simulink model "simulink_multiple_step_ODE_PID"  (R2023a)
settings: Solver=ode45  StartTime=0.0  StopTime=15000  RelTol=1e-3
libraries: slpidlib x1
settings Model: Creator=USER  LastModifiedBy=USER

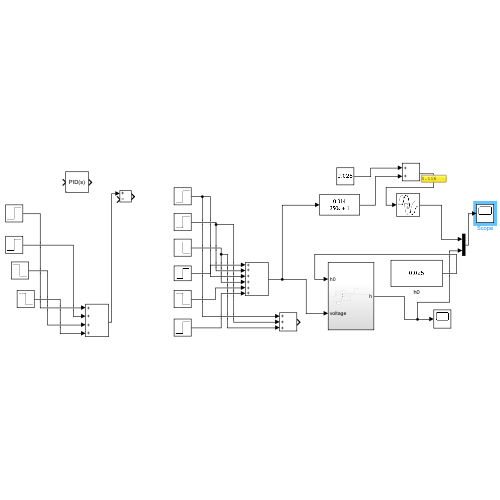
[thumbnail: Simulink's stored preview of the top-level diagram]
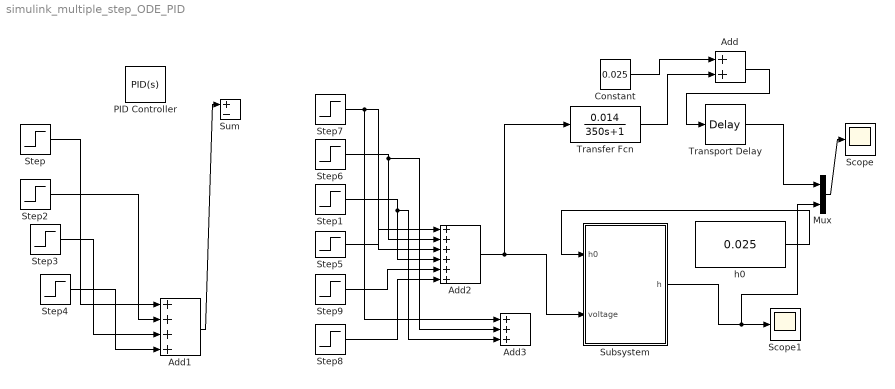
== system simulink_multiple_step_ODE_PID ==
  Add : Sum
  Add1 : Sum  Inputs=++++
  Add2 : Sum  Inputs=++++++
  Add3 : Sum  Inputs=+++
  Constant : Constant  Value=0.025
  Mux : Mux  Inputs=2
  PID Controller : slpidlib/PID Controller  Controller=PID  Form=Parallel  TimeDomain=Continuous-time  UseExternalTs=off  SampleTime=-1  IntegratorMethod=Forward Euler  FilterMethod=Forward Euler  ControllerParametersSource=internal  P=1  I=10  UseKiTs=off  D=0  N=100  UseFilter=on  TunerSelectOption=Transfer Function Based (PID Tuner App)  InitialConditionSource=internal  InitialConditionForIntegrator=0  InitialConditionForFilter=0  DifferentiatorICPrevScaledInput=0  ExternalReset=none  TrackingMode=off  Kt=1  LimitOutput=off  SatLimitsSource=internal  UpperSaturationLimit=inf  LowerSaturationLimit=-inf  LinearizeAsGain=on  AntiWindupMode=none  Kb=1  LimitIntegrator=off  UpperIntegratorSaturationLimit=inf  LowerIntegratorSaturationLimit=-inf  POutMin=[]  POutMax=[]  IOutMin=[]  IOutMax=[]  DOutMin=[]  DOutMax=[]  NOutMin=[]  NOutMax=[]  SumOutMin=[]  SumOutMax=[]  SaturationOutMin=[]  SaturationOutMax=[]  PParamMin=[]  PParamMax=[]  IParamMin=[]  IParamMax=[]  DParamMin=[]  DParamMax=[]  NParamMin=[]  NParamMax=[]  KbParamMin=[]  KbParamMax=[]  KtParamMin=[]  KtParamMax=[]  KbOutMin=[]  KbOutMax=[]  KtOutMin=[]  KtOutMax=[]  IntegratorOutMin=[]  IntegratorOutMax=[]  FilterOutMin=[]  FilterOutMax=[]  SumI1OutMin=[]  SumI1OutMax=[]  SumI2OutMin=[]  SumI2OutMax=[]  SumI3OutMin=[]  SumI3OutMax=[]  SumI4OutMin=[]  SumI4OutMax=[]  SumDOutMin=[]  SumDOutMax=[]  DifferentiatorOutMin=[]  DifferentiatorOutMax=[]  FilterDiffOutCoefMin=[]  FilterDiffOutCoefMax=[]  ReciprocalOutMin=[]  ReciprocalOutMax=[]  SumDenOutMin=[]  SumDenOutMax=[]  SumNumOutMin=[]  SumNumOutMax=[]  DivideOutMin=[]  DivideOutMax=[]  UdiffTsProdOutMin=[]  UdiffTsProdOutMax=[]  NTsProdOutMin=[]  NTsProdOutMax=[]  UintegralTsProdOutMin=[]  UintegralTsProdOutMax=[]  UngainTsProdOutMin=[]  UngainTsProdOutMax=[]  ClampingZeroOutDataTypeStr=Inherit: Inherit via back propagation  ClampingZeroOutMin=[]  ClampingZeroOutMax=[]  FilterDenConstantOutDataTypeStr=Inherit: Inherit via back propagation  FilterDenConstantOutMin=[]  FilterDenConstantOutMax=[]  PCopyOutDataTypeStr=Inherit: Inherit via back propagation  PCopyOutMin=[]  PCopyOutMax=[]  NCopyOutDataTypeStr=Inherit: Inherit via back propagation  NCopyOutMin=[]  NCopyOutMax=[]  IntegratorContinuousStateAttributes=''  IntegratorStateMustResolveToSignalObject=off  IntegratorRTWStateStorageClass=Auto  FilterContinuousStateAttributes=''  FilterStateMustResolveToSignalObject=off  FilterRTWStateStorageClass=Auto  ParallelPVariant=InternalParameters  IdealPVariant=Disabled  IVariant=InternalParameters  DVariant=InternalParameters  IntegratorVariant=Continuous  SatVariant=Disabled  AWVariant=Passthrough  PCopyVariant=Disabled  TRVariant=Disabled  FdbkBlocksVariant=Forward  IdealPFdbkVariant=Disabled  SatFdbkVariant=Disabled  DerivativeFilterVariant=ContFilter  NVariant=InternalParameters  NCopyVariant=Disabled  FilterICVariant=InternalICsFilter  IntegratorICVariant=InternalICs  ExternalResetVariant=Disabled  TRSumVariant=Passthrough  SumFdbkVariant=Disabled  SumVariant=Sum_PID  TsampFilterVariant=InternalTs  TsampNgainVariant=Passthrough  TsampIntegralVariant=Disabled_SignalSpec  ExternalSaturationOutDataTypeStr=Inherit: Same as second input
  Scope : Scope
  Scope1 : Scope
  Step : Step  Time=100  Before=0.025  After=0.05  SampleTime=0.01
  Step1 : Step  Time=7000  After=-3  SampleTime=0.01
  Step2 : Step  Time=2500  After=0.05  SampleTime=0
  Step3 : Step  Time=5000  After=-0.02  SampleTime=0
  Step4 : Step  Time=7500  After=-0.03  SampleTime=0
  Step5 : Step  Time=8500  After=2  SampleTime=0.01
  Step6 : Step  Time=4000  After=2  SampleTime=0.01
  Step7 : Step  Time=0  After=5  SampleTime=0.01
  Step8 : Step  Time=12500  After=4  SampleTime=0.01
  Step9 : Step  Time=10000  After=-3.5  SampleTime=0.01
  Subsystem : Subsystem
  Sum : Sum  Inputs=+-
  Transfer Fcn : TransferFcn  Numerator=[0.014]  Denominator=[350 1]
  Transport Delay : TransportDelay  DelayTime=100  InitialOutput=0.025
  h0 : Constant  Value=0.025
  wires:
  Subsystem/1(h) -> Mux/2, Scope1/1
  Step/1 -> Add1/1
  Step2/1 -> Add1/2
  Step3/1 -> Add1/3
  Step4/1 -> Add1/4
  Add1/1 -> Sum/1
  h0/1 -> Subsystem/1(h0)
  Step1/1 -> Add3/3, Add2/4
  Step5/1 -> Add2/1
  Step9/1 -> Add2/5
  Step8/1 -> Add2/6
  Step7/1 -> Add3/1, Add2/3
  Step6/1 -> Add3/2, Add2/2
  Mux/1 -> Scope/1
  Constant/1 -> Add/1
  Transfer Fcn/1 -> Add/2
  Add/1 -> Transport Delay/1
  Transport Delay/1 -> Mux/1
  Add2/1 -> Transfer Fcn/1, Subsystem/2(voltage)

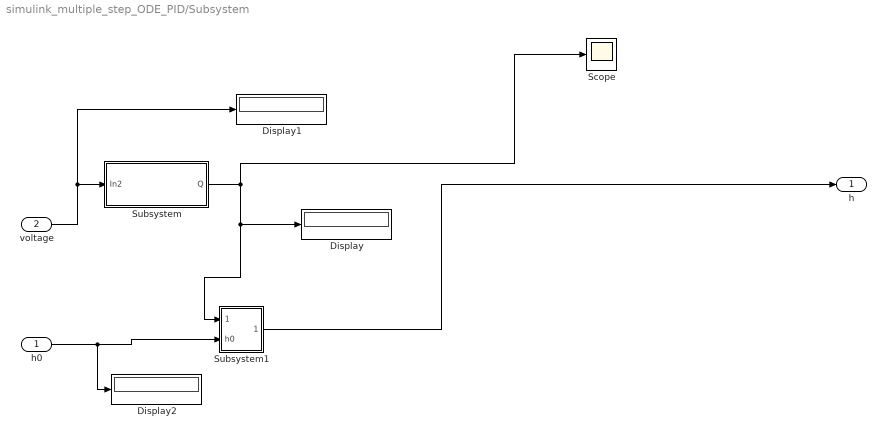
== system simulink_multiple_step_ODE_PID/Subsystem ==
  h0 : Inport
  voltage : Inport  Port=2
  Display : Display
  Display1 : Display
  Display2 : Display
  Scope : Scope
  Subsystem : Subsystem
  Subsystem1 : Subsystem
  h : Outport
  wires:
  Subsystem/1(Q) -> Subsystem1/1(In1), Display/1, Scope/1
  h0/1 -> Display2/1, Subsystem1/2(h0)
  Subsystem1/1(Out1) -> h/1
  voltage/1 -> Display1/1, Subsystem/1(In2)

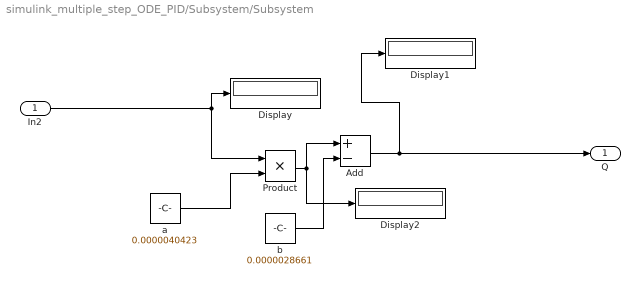
== system simulink_multiple_step_ODE_PID/Subsystem/Subsystem ==
  In2 : Inport
  Add : Sum  Inputs=+-
  Display : Display
  Display1 : Display
  Display2 : Display
  Product : Product
  a : Constant  Value=0.0000040423
  b : Constant  Value=0.0000028661
  Q : Outport
  wires:
  a/1 -> Product/2
  Product/1 -> Add/1, Display2/1
  b/1 -> Add/2
  Add/1 -> Display1/1, Q/1
  In2/1 -> Product/1, Display/1

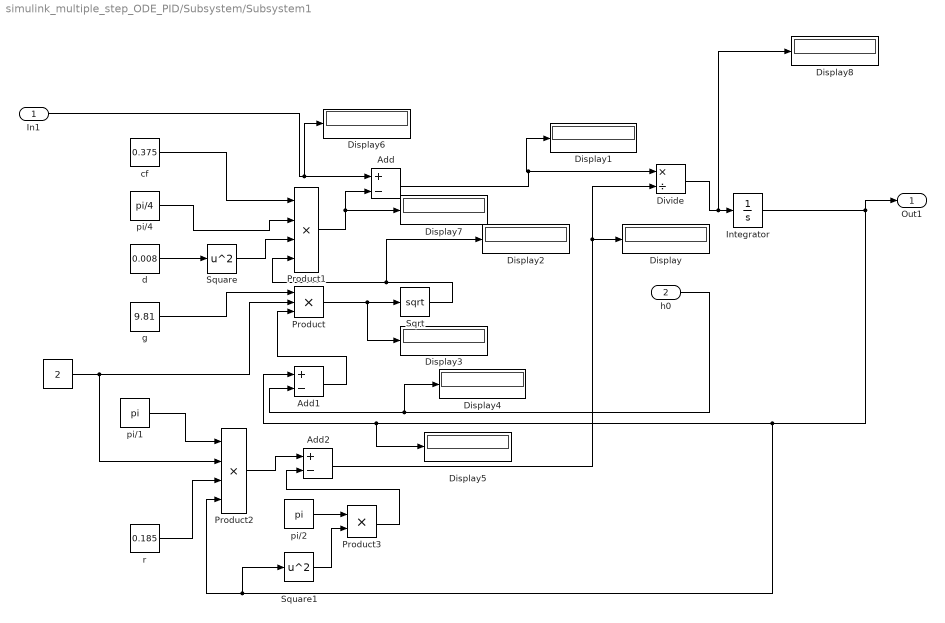
== system simulink_multiple_step_ODE_PID/Subsystem/Subsystem1 ==
  In1 : Inport
  h0 : Inport  Port=2
  " " : Constant  Value=2
  Add : Sum  Inputs=+-
  Add1 : Sum  Inputs=+-
  Add2 : Sum  Inputs=+-
  Display{,1..8} (9 alike) : Display
  Divide : Product  Inputs=*/
  Integrator : Integrator  InitialCondition=0.025
  Product : Product  Inputs=3
  Product1 : Product  Inputs=4
  Product2 : Product  Inputs=4
  Product3 : Product
  Sqrt : Sqrt
  Square : Math  Operator=square
  Square1 : Math  Operator=square
  cf : Constant  Value=0.375
  d : Constant  Value=0.008
  g : Constant  Value=9.81
  pi/1 : Constant  Value=pi
  pi/2 : Constant  Value=pi
  pi/4 : Constant  Value=pi/4
  r : Constant  Value=0.185
  Out1 : Outport
  wires:
  pi/1/1 -> Product2/1
  Add1/1 -> Product/3
  Product1/1 -> Display7/1, Add/2
  Divide/1 -> Display8/1, Integrator/1
  Product3/1 -> Add2/2
  " "/1 -> Product2/2, Product/2
  cf/1 -> Product1/1
  r/1 -> Product2/3
  Sqrt/1 -> Display2/1, Product1/4
  Square/1 -> Product1/3
  Product2/1 -> Add2/1
  pi/4/1 -> Product1/2
  h0/1 -> Display4/1, Add1/2
  g/1 -> Product/1
  d/1 -> Square/1
  Product/1 -> Display3/1, Sqrt/1
  Add/1 -> Divide/1, Display1/1
  Square1/1 -> Product3/2
  In1/1 -> Add/1, Display6/1
  pi/2/1 -> Product3/1
  Add2/1 -> Display/1, Divide/2
  Integrator/1 -> Out1/1, Product2/4, Square1/1, Display5/1, Add1/1
